simulink model "sim_env_falling_leaf_linear"  (R2023b)
settings: Solver=ode113  StartTime=0.0  StopTime=20  RelTol=1e-3
model workspace (MAT data in the model file):
  ail_0 = -0.0765
undefined symbols (not defined in the file or in its folder): A, B, C, D, x0
settings Model: Creator=ac140857  LastModifiedBy=fabioschneider
settings DebuggingCC: AlgebraicLoopMsg=none  ModelReferenceExtraNoncontSigs=none

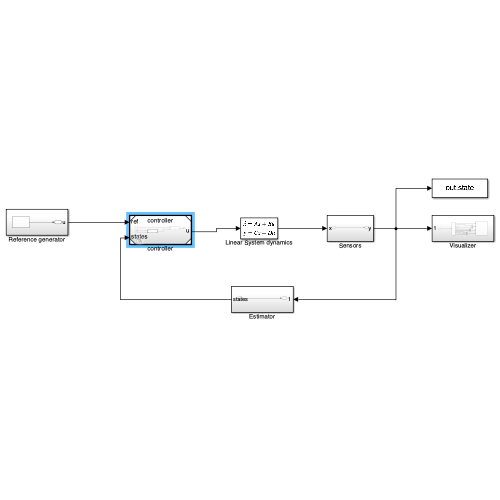
[thumbnail: Simulink's stored preview of the top-level diagram]
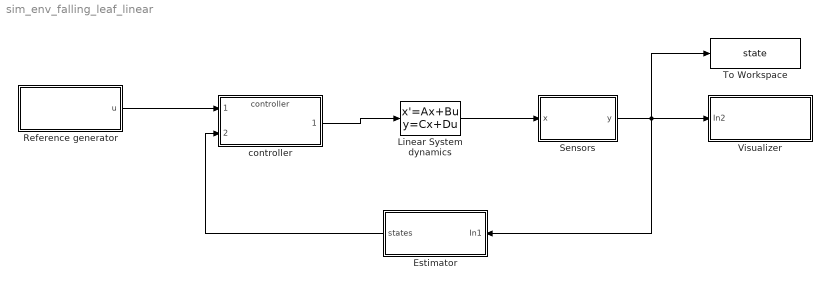
== system sim_env_falling_leaf_linear ==
  Estimator : Subsystem
  Linear System dynamics : StateSpace  A=A  B=B  C=C  D=D  InitialCondition=x0
  Reference generator : Subsystem
  Sensors : Subsystem
  To Workspace : ToWorkspace  VariableName=state  SaveFormat=Timeseries  SampleTime=-1
  Visualizer : Subsystem
  controller : ModelReference  ModelNameDialog=controller.slx  SimulationMode=Normal  ModelReferenceVersion=1.2
  wires:
  Reference generator/1(u) -> controller/1
  Estimator/1(states) -> controller/2
  Sensors/1(y) -> To Workspace/1, Visualizer/1(In2), Estimator/1(In1)
  controller/1 -> Linear System dynamics/1
  Linear System dynamics/1 -> Sensors/1(x)

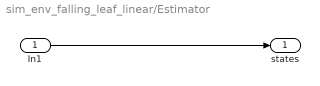
== system sim_env_falling_leaf_linear/Estimator ==
  In1 : Inport
  states : Outport
  wires:
  In1/1 -> states/1

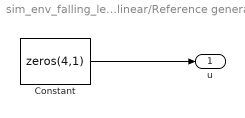
== system sim_env_falling_leaf_linear/Reference generator ==
  Constant : Constant  Value=zeros(4,1)  SampleTime=-1
  u : Outport
  wires:
  Constant/1 -> u/1

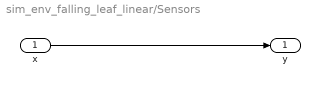
== system sim_env_falling_leaf_linear/Sensors ==
  x : Inport
  y : Outport
  wires:
  x/1 -> y/1

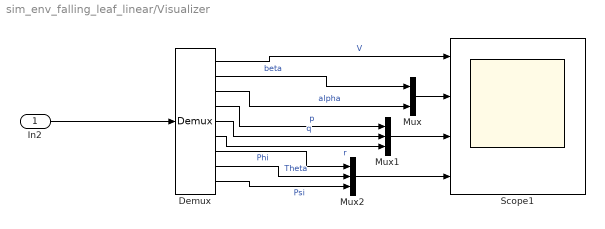
== system sim_env_falling_leaf_linear/Visualizer ==
  In2 : Inport
  Demux : Demux  Outputs=9
  Mux : Mux  Inputs=2
  Mux1 : Mux  Inputs=3
  Mux2 : Mux  Inputs=3
  Scope1 : Scope  NumInputPorts=4
  wires:
  In2/1 -> Demux/1
  Demux/6 -> Mux1/3  "r"
  Demux/5 -> Mux1/2  "q"
  Demux/4 -> Mux1/1  "p"
  Demux/8 -> Mux2/2  "Theta"
  Demux/7 -> Mux2/1  "Phi"
  Demux/2 -> Mux/1  "beta"
  Demux/1 -> Scope1/1  "V"
  Mux/1 -> Scope1/2
  Demux/3 -> Mux/2  "alpha"
  Mux2/1 -> Scope1/4
  Demux/9 -> Mux2/3  "Psi"
  Mux1/1 -> Scope1/3
